simulink model "sampleModel200"  (R2021b)
settings: Solver=VariableStepAuto  StartTime=0.0  StopTime=10.0  RelTol=1e-3
undefined symbols (not defined in the file or in its folder): Newton, Raphson
libraries: simulink x4
settings Model: Creator=user  LastModifiedBy=user

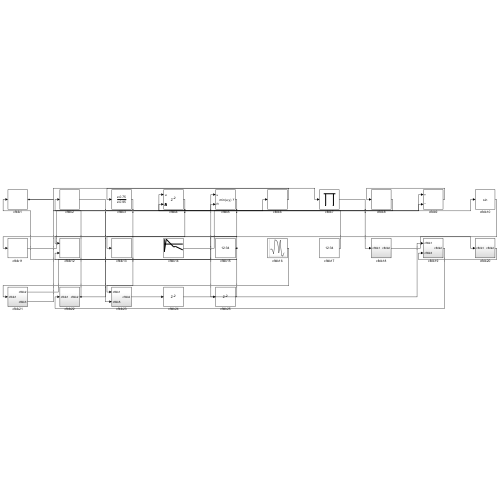
[thumbnail: Simulink's stored preview of the top-level diagram]
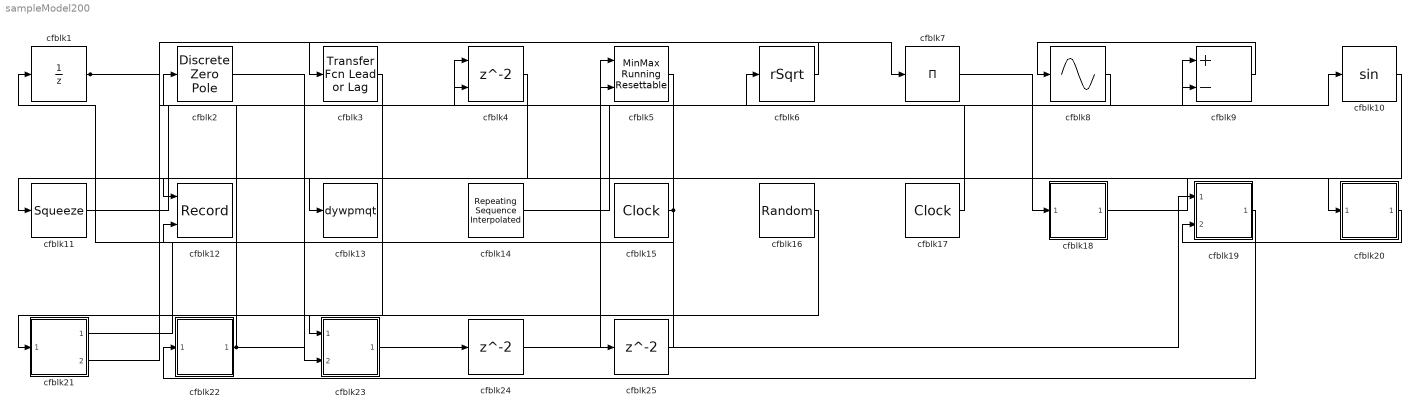
== system sampleModel200 ==
  cfblk1 : UnitDelay  HasFrameUpgradeWarning=on
  cfblk10 : Trigonometry
  cfblk11 : Squeeze
  cfblk12 : Record  FileSettingsInternal="{\"entries\":[{\"content\":{\"excelSettings\":{\"content\":{},\"type\":\"Streamout.ExcelSettings\"}},\"type\":\"Streamout.FileSettingStorage\",\"uuid\":\"792bf4ae-df5f-4a02-8cd9-bdcd44b156f6\"}],\"packageUris\":[\"http://schema.mathworks.com/mf0/streamout_blocks/R2020a\"],\"version\":\"1.0\"}"  Layout=[1 1]  SignalsInternal="{\"entries\":[{\"content\":{\"signals\":[{\"content\":{\"blockPath\":[\"sampleModel200/cfblk12\"],\"channel\":[],\"dimensions\":[1],\"domain\":\"sampleModel200/cfblk12\",\"lineColor\":\"#a2142f\",\"plots\":[1],\"port\":1,\"sid\":[\"\"],\"signalID\":7649,\"signalName\":\"cfblk3\"},\"type\":\"RecordBlkView.Signal\",\"uuid\":\"51a90d37-c1cf-4aff-97b9-1f3611509108\"},{\"content\":{\"blockPath\":[\"sampleModel200/cfblk12\"],\"channel\":[],\"dimensions\":[1],\"domain\":\"sampleModel200/cfblk12\",\"lineColor\":\"#139fff\",\"plots\":[1],\"port\":2,\"sid\":[\"\"],\"signalID\":7653,\"signalName\":\"cfblk15\"},\"type\":\"RecordBlkView.Signal\",\"uuid\":\"2278662f-4324-4c25-a22a-e30aa41c0c8f\"}]},\"type\":\"RecordBlkView.InputSignals\",\"uuid\":\"be1db6e8-9c30-458d-96b7-b90e03485ee9\"}],\"packageUris\":[\"http://schema.mathworks.com/mf0/streamout_blocks/R2020a\"],\"version\":\"1.0\"}"  VisualizationBindings="{\"xyplotplugin\":{\"info\":[{\"series\":[{\"bindingParametersList\":[{\"parameter\":\"X-Axis\",\"signalID\":7649,\"signalName\":\"cfblk3\"},{\"parameter\":\"Y-Axis\",\"signalID\":7653,\"signalName\":\"cfblk15\"}],\"seriesID\":1125}],\"subplotID\":1}]}}"  CompatibilityTag=XY
  cfblk13 : ToWorkspace  VariableName=dywpmqt  SaveFormat=Timeseries  SampleTime=-1
  cfblk14 : simulink/Sources/Repeating Sequence Interpolated  OutValues=[-759072475.643310, 482186398.603512, -297885325.500330, -221444817.303025, -587161699.163116]  TimeValues=[0 0.1 0.5 0.6 1].'  LookUpMeth=Use Input Below  tsamp=0.01  OutMin=[]  OutMax=[]  OutDataTypeStr=double  OutputDataTypeScalingMode=double  OutDataType=fixdt(0,8)  OutScaling=2^-10
  cfblk15 : DigitalClock
  cfblk16 : RandomNumber  Mean=[6390.487041]  Variance=[16438.141361]  Seed=[695413939.000000]  SampleTime=0.1
  cfblk17 : DigitalClock
  cfblk18 : Subsystem
  cfblk19 : Subsystem
  cfblk2 : DiscreteZeroPole  Poles=[0 0.5]  Gain=1
  cfblk20 : Subsystem
  cfblk21 : Subsystem
  cfblk22 : Subsystem
  cfblk23 : Subsystem
  cfblk24 : Delay  SampleTime=1
  cfblk25 : Delay  SampleTime=1
  cfblk3 : simulink/Discrete/Transfer Fcn Lead or Lag  PoleZ=0.95  ZeroZ=0.75  ICPrevOutput=0.0  ICPrevInput=0.0  DoSatur=off
      settings: SourceProductBaseCode=SL
  cfblk4 : Delay  ShowEnablePort=on  SampleTime=1
      settings: InputPortMap=u0,e6
  cfblk5 : simulink/Math Operations/MinMax Running Resettable  Function=min  vinit=0.0
  cfblk6 : Sqrt  Operator=rSqrt  AlgorithmType=Newton-Raphson  SaturateOnIntegerOverflow=on
  cfblk7 : Product  Inputs=*
  cfblk8 : Sin  TimeSource=Use external signal  SampleTime=0
  cfblk9 : Sum  Inputs=+-
  wires:
  cfblk18/1(cfblk2) -> cfblk20/1(cfblk1)
  cfblk15/1 -> cfblk13/1, cfblk12/2
  cfblk11/1 -> cfblk10/1
  cfblk16/1 -> cfblk21/1(cfblk1)
  cfblk5/1 -> cfblk23/1(cfblk1)
  cfblk4/1 -> cfblk11/1
  cfblk19/1(cfblk2) -> cfblk22/1(cfblk1)
  cfblk21/1(cfblk2) -> cfblk5/1
  cfblk22/1(cfblk2) -> cfblk2/1, cfblk9/2
  cfblk20/1(cfblk2) -> cfblk19/2(cfblk3)
  cfblk17/1 -> cfblk4/1
  cfblk9/1 -> cfblk8/1
  cfblk1/1 -> cfblk7/1, cfblk5/2
  cfblk21/2(cfblk3) -> cfblk6/1
  cfblk3/1 -> cfblk12/1
  cfblk2/1 -> cfblk23/2(cfblk5)
  cfblk7/1 -> cfblk18/1(cfblk1)
  cfblk14/1 -> cfblk9/1
  cfblk6/1 -> cfblk3/1
  cfblk8/1 -> cfblk4/2
  cfblk23/1(cfblk2) -> cfblk24/1
  cfblk24/1 -> cfblk19/1(cfblk1)
  cfblk10/1 -> cfblk25/1
  cfblk25/1 -> cfblk1/1

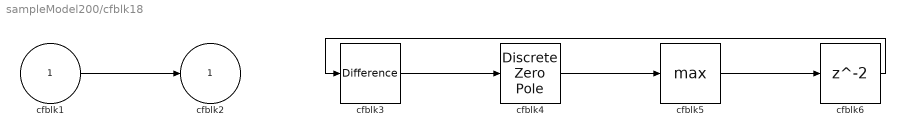
== system sampleModel200/cfblk18 ==
  cfblk1 : Inport
  cfblk3 : simulink/Discrete/Difference  ICPrevInput=0.0  OutMin=[]  OutMax=[]  OutDataTypeStr=Inherit: Inherit via back propagation  OutDataType=fixdt(1, 16)  OutScaling=2^-10  DoSatur=off
  cfblk4 : DiscreteZeroPole  Poles=[0 0.5]  Gain=1
  cfblk5 : MinMax  Function=max
  cfblk6 : Delay  SampleTime=1
  cfblk2 : Outport
  wires:
  cfblk3/1 -> cfblk4/1
  cfblk1/1 -> cfblk2/1
  cfblk4/1 -> cfblk5/1
  cfblk5/1 -> cfblk6/1
  cfblk6/1 -> cfblk3/1

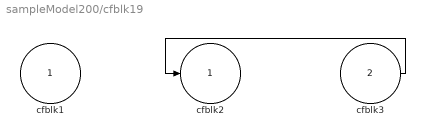
== system sampleModel200/cfblk19 ==
  cfblk1 : Inport
  cfblk3 : Inport  Port=2
  cfblk2 : Outport
  wires:
  cfblk3/1 -> cfblk2/1

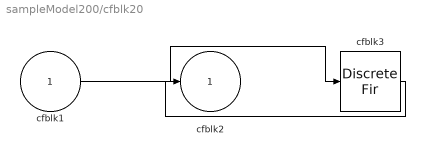
== system sampleModel200/cfblk20 ==
  cfblk1 : Inport
  cfblk3 : DiscreteFir  SampleTime=1
  cfblk2 : Outport
  wires:
  cfblk1/1 -> cfblk3/1
  cfblk3/1 -> cfblk2/1

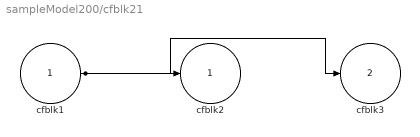
== system sampleModel200/cfblk21 ==
  cfblk1 : Inport
  cfblk2 : Outport
  cfblk3 : Outport  Port=2
  wires:
  cfblk1/1 -> cfblk3/1, cfblk2/1

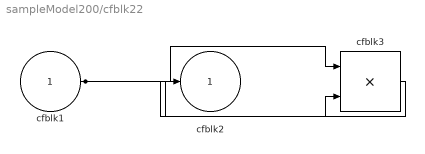
== system sampleModel200/cfblk22 ==
  cfblk1 : Inport
  cfblk3 : Product
  cfblk2 : Outport
  wires:
  cfblk1/1 -> cfblk3/1, cfblk3/2
  cfblk3/1 -> cfblk2/1

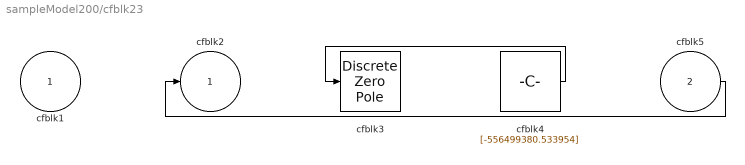
== system sampleModel200/cfblk23 ==
  cfblk1 : Inport
  cfblk5 : Inport  Port=2
  cfblk3 : DiscreteZeroPole  Poles=[0 0.5]  Gain=1
  cfblk4 : Constant  Value=[-556499380.533954]  SampleTime=1
  cfblk2 : Outport
  wires:
  cfblk4/1 -> cfblk3/1
  cfblk5/1 -> cfblk2/1
